simulink model "DALv3"  (R2021b)
settings: Solver=VariableStepAuto  StartTime=0.0  StopTime=10.0  RelTol=1e-3
values from neighbouring files (symbols this model uses):
  Beam_Mod = 1013.21*5/1023*ones(n_sensors,1)    [DAL_Declarations.m]
  N_B = [1 0 0; -1 0 0 ... (first row only)    [DAL_Declarations.m]
  Theta_rel = 0    [DAL_Declarations.m]
undefined symbols (not defined in the file or in its folder): magnitude
libraries: slpidlib x1
settings Model: Creator=Andrea  LastModifiedBy=Andrea

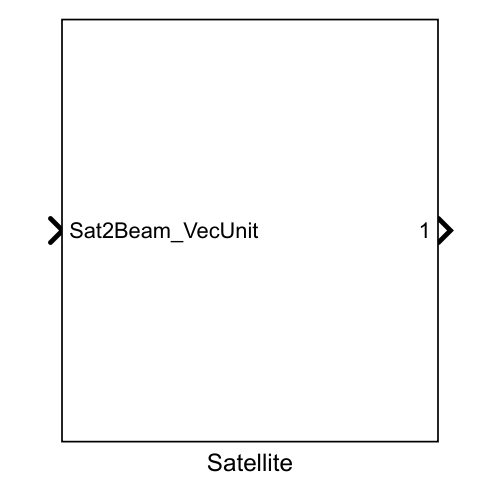
[thumbnail: Simulink's stored preview of the top-level diagram]
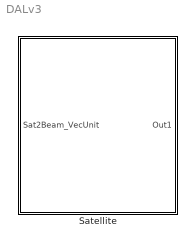
== system DALv3 ==
  Satellite : Subsystem

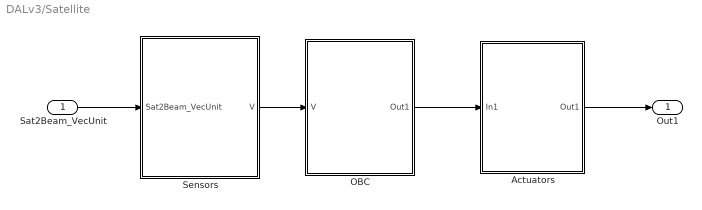
== system DALv3/Satellite ==
  Sat2Beam_VecUnit : Inport
  Actuators : Subsystem
  OBC : Subsystem
  Sensors : Subsystem
  Out1 : Outport
  wires:
  Sat2Beam_VecUnit/1 -> Sensors/1(Sat2Beam_VecUnit)
  OBC/1(Out1) -> Actuators/1(In1)
  Sensors/1(V) -> OBC/1(V)
  Actuators/1(Out1) -> Out1/1

== system DALv3/Satellite/Actuators ==
  In1 : Inport
  Out1 : Outport
  wires:
  In1/1 -> Out1/1

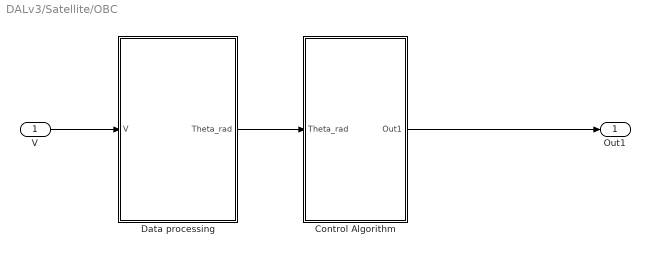
== system DALv3/Satellite/OBC ==
  V : Inport
  Control Algorithm : Subsystem
  Data processing : Subsystem
  Out1 : Outport
  wires:
  V/1 -> Data processing/1(V)
  Data processing/1(Theta_rad) -> Control Algorithm/1(Theta_rad)
  Control Algorithm/1(Out1) -> Out1/1

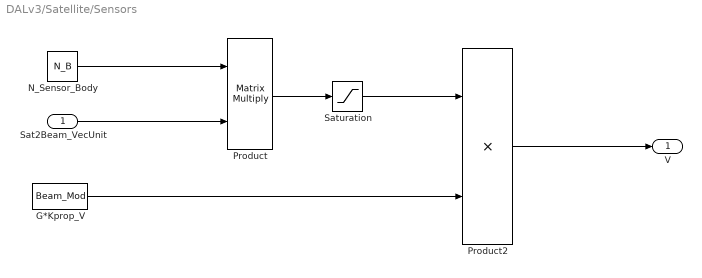
== system DALv3/Satellite/Sensors ==
  Sat2Beam_VecUnit : Inport  OutDataTypeStr=double
  G*Kprop_V : Constant  Value=Beam_Mod
  N_Sensor_Body : Constant  Value=N_B
  Product : Product  Multiplication=Matrix(*)
  Product2 : Product
  Saturation : Saturate  UpperLimit=1  LowerLimit=0
  V : Outport
  wires:
  Product/1 -> Saturation/1
  Sat2Beam_VecUnit/1 -> Product/2
  N_Sensor_Body/1 -> Product/1
  Saturation/1 -> Product2/1
  G*Kprop_V/1 -> Product2/2
  Product2/1 -> V/1

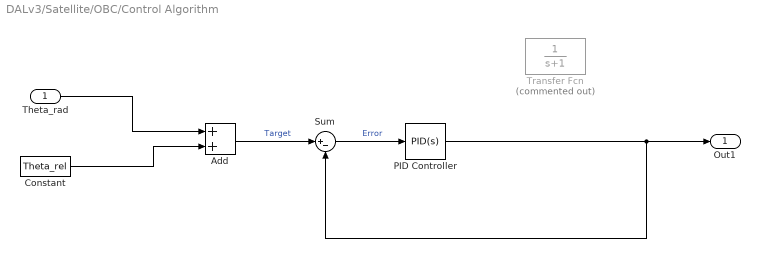
== system DALv3/Satellite/OBC/Control Algorithm ==
  Theta_rad : Inport
  Add : Sum
  Constant : Constant  Value=Theta_rel
  PID Controller : slpidlib/PID Controller  Controller=PID  Form=Parallel  TimeDomain=Continuous-time  UseExternalTs=off  SampleTime=-1  IntegratorMethod=Forward Euler  FilterMethod=Forward Euler  ControllerParametersSource=internal  P=1  I=1  D=0  UseFilter=on  N=100  TunerSelectOption=Transfer Function Based (PID Tuner App)  InitialConditionSource=internal  InitialConditionForIntegrator=0  InitialConditionForFilter=0  DifferentiatorICPrevScaledInput=0  ExternalReset=none  TrackingMode=off  Kt=1  LimitOutput=off  SatLimitsSource=internal  UpperSaturationLimit=inf  LowerSaturationLimit=-inf  LinearizeAsGain=on  AntiWindupMode=none  Kb=1  POutMin=[]  POutMax=[]  IOutMin=[]  IOutMax=[]  DOutMin=[]  DOutMax=[]  NOutMin=[]  NOutMax=[]  SumOutMin=[]  SumOutMax=[]  SaturationOutMin=[]  SaturationOutMax=[]  PParamMin=[]  PParamMax=[]  IParamMin=[]  IParamMax=[]  DParamMin=[]  DParamMax=[]  NParamMin=[]  NParamMax=[]  KbParamMin=[]  KbParamMax=[]  KtParamMin=[]  KtParamMax=[]  KbOutMin=[]  KbOutMax=[]  KtOutMin=[]  KtOutMax=[]  IntegratorOutMin=[]  IntegratorOutMax=[]  FilterOutMin=[]  FilterOutMax=[]  SumI1OutMin=[]  SumI1OutMax=[]  SumI2OutMin=[]  SumI2OutMax=[]  SumI3OutMin=[]  SumI3OutMax=[]  SumI4OutMin=[]  SumI4OutMax=[]  SumDOutMin=[]  SumDOutMax=[]  DifferentiatorOutMin=[]  DifferentiatorOutMax=[]  FilterDiffOutCoefMin=[]  FilterDiffOutCoefMax=[]  ReciprocalOutMin=[]  ReciprocalOutMax=[]  SumDenOutMin=[]  SumDenOutMax=[]  SumNumOutMin=[]  SumNumOutMax=[]  DivideOutMin=[]  DivideOutMax=[]  UdiffTsProdOutMin=[]  UdiffTsProdOutMax=[]  NTsProdOutMin=[]  NTsProdOutMax=[]  UintegralTsProdOutMin=[]  UintegralTsProdOutMax=[]  UngainTsProdOutMin=[]  UngainTsProdOutMax=[]  IntegratorContinuousStateAttributes=''  IntegratorStateMustResolveToSignalObject=off  IntegratorRTWStateStorageClass=Auto  FilterContinuousStateAttributes=''  FilterStateMustResolveToSignalObject=off  FilterRTWStateStorageClass=Auto  ParallelPVariant=InternalParameters  IdealPVariant=Disabled  IVariant=InternalParameters  DVariant=InternalParameters  IntegratorVariant=Continuous  SatVariant=Disabled  AWVariant=Passthrough  PCopyVariant=Disabled  TRVariant=Disabled  FdbkBlocksVariant=Forward  IdealPFdbkVariant=Disabled  SatFdbkVariant=Disabled  DerivativeFilterVariant=ContFilter  NVariant=InternalParameters  NCopyVariant=Disabled  FilterICVariant=InternalICsFilter  IntegratorICVariant=InternalICs  ExternalResetVariant=Disabled  TRSumVariant=Passthrough  SumFdbkVariant=Disabled  SumVariant=Sum_PID  TsampFilterVariant=InternalTs  TsampNgainVariant=Passthrough  TsampIntegralVariant=Passthrough  ExternalSaturationOutDataTypeStr=Inherit: Same as second input
  Sum : Sum  Inputs=|+-
  Transfer Fcn : TransferFcn  Commented=on  Denominator=[1 1]
  Out1 : Outport
  wires:
  Theta_rad/1 -> Add/1
  PID Controller/1 -> Sum/2, Out1/1
  Constant/1 -> Add/2
  Add/1 -> Sum/1  "Target"
  Sum/1 -> PID Controller/1  "Error"

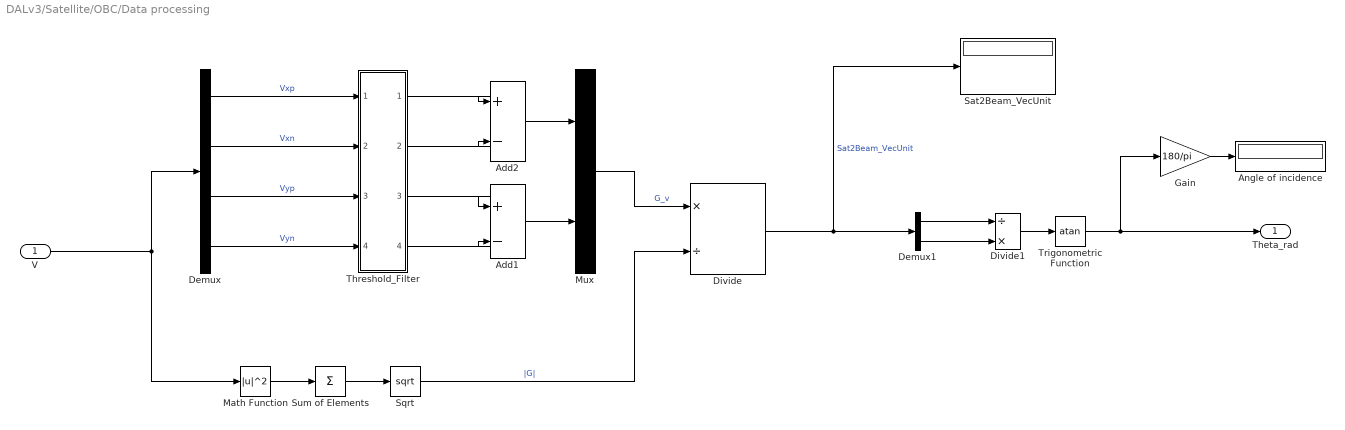
== system DALv3/Satellite/OBC/Data processing ==
  V : Inport
  Add1 : Sum  Inputs=+|-
  Add2 : Sum  Inputs=+|-
  Angle of incidence : Display
  Demux : Demux
  Demux1 : Demux  Outputs=2
  Divide : Product  Inputs=*/
  Divide1 : Product  Inputs=/*
  Gain : Gain  Gain=180/pi
  Math Function : Math  Operator=magnitude^2  OutputSignalType=real  SaturateOnIntegerOverflow=on
  Mux : Mux  Inputs=2
  Sat2Beam_VecUnit : Display
  Sqrt : Sqrt  SaturateOnIntegerOverflow=on
  Sum of Elements : Sum  Inputs=+
  Threshold_Filter : Subsystem
  Trigonometric Function : Trigonometry  Operator=atan
  Theta_rad : Outport
  wires:
  Threshold_Filter/3(Out3) -> Add1/1
  Threshold_Filter/1(Out1) -> Add2/1
  Threshold_Filter/2(Out2) -> Add2/2
  Demux/4 -> Threshold_Filter/4(Vyn)  "Vyn"
  Demux/2 -> Threshold_Filter/2(Vxn)  "Vxn"
  Demux/1 -> Threshold_Filter/1(Vxp)  "Vxp"
  Demux/3 -> Threshold_Filter/3(Vyp)  "Vyp"
  Threshold_Filter/4(Out4) -> Add1/2
  Math Function/1 -> Sum of Elements/1
  Trigonometric Function/1 -> Gain/1, Theta_rad/1
  Divide1/1 -> Trigonometric Function/1
  Divide/1 -> Demux1/1, Sat2Beam_VecUnit/1  "Sat2Beam_VecUnit"
  Add2/1 -> Mux/1
  Add1/1 -> Mux/2
  Demux1/1 -> Divide1/1
  Mux/1 -> Divide/1  "G_v"
  V/1 -> Math Function/1, Demux/1
  Sum of Elements/1 -> Sqrt/1
  Demux1/2 -> Divide1/2
  Gain/1 -> Angle of incidence/1
  Sqrt/1 -> Divide/2  "|G|"

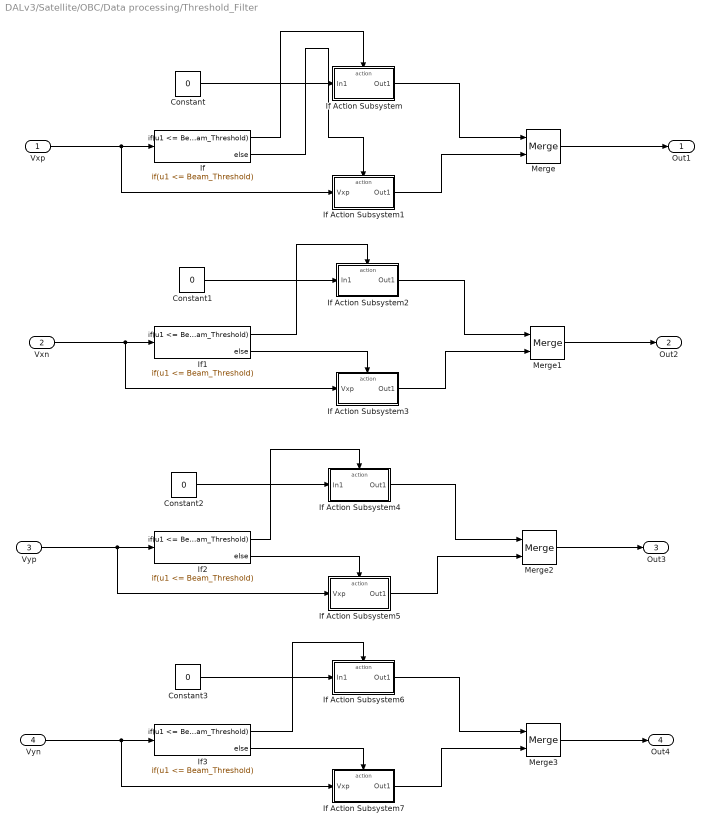
== system DALv3/Satellite/OBC/Data processing/Threshold_Filter ==
  Vxp : Inport
  Vxn : Inport  Port=2
  Vyp : Inport  Port=3
  Vyn : Inport  Port=4
  Constant{,1..3} (4 alike) : Constant  Value=0
  If{,1..3} (4 alike) : If  IfExpression=u1 <= Beam_Threshold
  If Action Subsystem : Subsystem  TreatAsAtomicUnit=on
  If Action Subsystem1 : Subsystem  TreatAsAtomicUnit=on
  If Action Subsystem2 : Subsystem  TreatAsAtomicUnit=on
  If Action Subsystem3 : Subsystem  TreatAsAtomicUnit=on
  If Action Subsystem4 : Subsystem  TreatAsAtomicUnit=on
  If Action Subsystem5 : Subsystem  TreatAsAtomicUnit=on
  If Action Subsystem6 : Subsystem  TreatAsAtomicUnit=on
  If Action Subsystem7 : Subsystem  TreatAsAtomicUnit=on
  Merge{,1..3} (4 alike) : Merge
  Out1 : Outport
  Out2 : Outport  Port=2
  Out3 : Outport  Port=3
  Out4 : Outport  Port=4
  wires:
  Vxp/1 -> If Action Subsystem1/1(Vxp), If/1
  If/1 -> If Action Subsystem/Action
  If Action Subsystem/1(Out1) -> Merge/1
  If/2 -> If Action Subsystem1/Action
  If Action Subsystem1/1(Out1) -> Merge/2
  Merge/1 -> Out1/1
  Constant/1 -> If Action Subsystem/1(In1)
  If Action Subsystem3/1(Out1) -> Merge1/2
  Constant1/1 -> If Action Subsystem2/1(In1)
  If1/1 -> If Action Subsystem2/Action
  Vxn/1 -> If1/1, If Action Subsystem3/1(Vxp)
  If Action Subsystem2/1(Out1) -> Merge1/1
  If1/2 -> If Action Subsystem3/Action
  Merge1/1 -> Out2/1
  Vyp/1 -> If2/1, If Action Subsystem5/1(Vxp)
  If2/2 -> If Action Subsystem5/Action
  If2/1 -> If Action Subsystem4/Action
  If Action Subsystem4/1(Out1) -> Merge2/1
  If Action Subsystem5/1(Out1) -> Merge2/2
  Constant2/1 -> If Action Subsystem4/1(In1)
  Merge2/1 -> Out3/1
  Vyn/1 -> If3/1, If Action Subsystem7/1(Vxp)
  Merge3/1 -> Out4/1
  If Action Subsystem7/1(Out1) -> Merge3/2
  If3/2 -> If Action Subsystem7/Action
  If Action Subsystem6/1(Out1) -> Merge3/1
  Constant3/1 -> If Action Subsystem6/1(In1)
  If3/1 -> If Action Subsystem6/Action

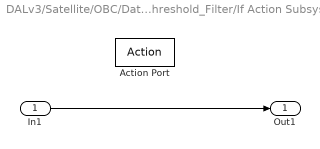
== system DALv3/Satellite/OBC/Data processing/Threshold_Filter/If Action Subsystem ==
  In1 : Inport
  Action Port : ActionPort
  Out1 : Outport
  wires:
  In1/1 -> Out1/1

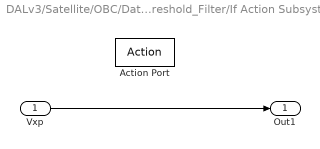
== system DALv3/Satellite/OBC/Data processing/Threshold_Filter/If Action Subsystem1 ==
  Vxp : Inport
  Action Port : ActionPort
  Out1 : Outport
  wires:
  Vxp/1 -> Out1/1

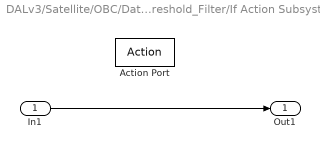
== system DALv3/Satellite/OBC/Data processing/Threshold_Filter/If Action Subsystem2 ==
  In1 : Inport
  Action Port : ActionPort
  Out1 : Outport
  wires:
  In1/1 -> Out1/1

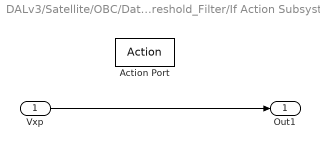
== system DALv3/Satellite/OBC/Data processing/Threshold_Filter/If Action Subsystem3 ==
  Vxp : Inport
  Action Port : ActionPort
  Out1 : Outport
  wires:
  Vxp/1 -> Out1/1

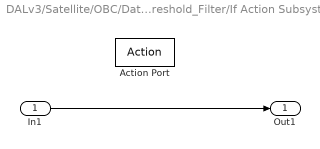
== system DALv3/Satellite/OBC/Data processing/Threshold_Filter/If Action Subsystem4 ==
  In1 : Inport
  Action Port : ActionPort
  Out1 : Outport
  wires:
  In1/1 -> Out1/1

== system DALv3/Satellite/OBC/Data processing/Threshold_Filter/If Action Subsystem5 ==
  Vxp : Inport
  Action Port : ActionPort
  Out1 : Outport
  wires:
  Vxp/1 -> Out1/1

== system DALv3/Satellite/OBC/Data processing/Threshold_Filter/If Action Subsystem6 ==
  In1 : Inport
  Action Port : ActionPort
  Out1 : Outport
  wires:
  In1/1 -> Out1/1

== system DALv3/Satellite/OBC/Data processing/Threshold_Filter/If Action Subsystem7 ==
  Vxp : Inport
  Action Port : ActionPort
  Out1 : Outport
  wires:
  Vxp/1 -> Out1/1
